simulink model "Dan_model3b"  (Simulink 7.8)
settings: Solver=ode45  StartTime=0.0  StopTime=10.0  RelTol=1e-3
values from neighbouring files (symbols this model uses):
  h = h_vec(i)    [ps7-task3.m]
  K = minreal(K_vec)    [ps7-task3.m]
libraries: cstblocks x2
settings Model: Creator=lifeofsacrifice  LastModifiedBy=Dan

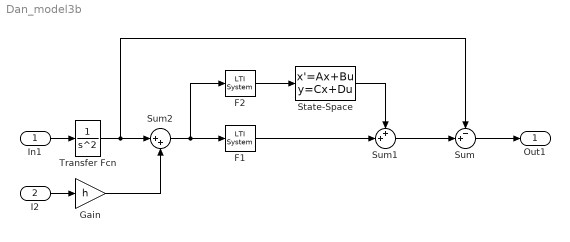
== system Dan_model3b ==
  In1 : Inport
  I2 : Inport  Port=2
  F1 : cstblocks/LTI System  sys=F1  IC=[]
  F2 : cstblocks/LTI System  sys=F2  IC=[]
  Gain : Gain  Gain=h
  State-Space : StateSpace  A=K.A  B=K.B  C=K.C  D=K.D
  Sum : Sum  Inputs=-+|
  Sum1 : Sum  Inputs=++|
  Sum2 : Sum  Inputs=|++
  Transfer Fcn : TransferFcn  Denominator=[1 0 0]
  Out1 : Outport
  wires:
  In1/1 -> Transfer Fcn/1
  Transfer Fcn/1 -> Sum2/1, Sum/1
  I2/1 -> Gain/1
  Gain/1 -> Sum2/2
  Sum2/1 -> F2/1, F1/1
  Sum/1 -> Out1/1
  Sum1/1 -> Sum/2
  F1/1 -> Sum1/2
  F2/1 -> State-Space/1
  State-Space/1 -> Sum1/1
